simulink model "Schema_Bloc_Instalatie"  (R2017b)
settings: Solver=VariableStepAuto  StartTime=0.0  StopTime=1000  RelTol=1e-3
values from neighbouring files (symbols this model uses):
  k = 0.035    [modelare.m]
  k11 = k2^2+4*(k-k3)*k1    (= 0.0890826)    [modelare.m]
  k12 = 4*(k-k3)*2    (= 0.2848)    [modelare.m]
  k13 = 2*(k-k3)    (= 0.0712)    [modelare.m]
  k2 = -0.015    [modelare.m]
settings Model: Creator=alinvoicu26  LastModifiedBy=alinvoicu26

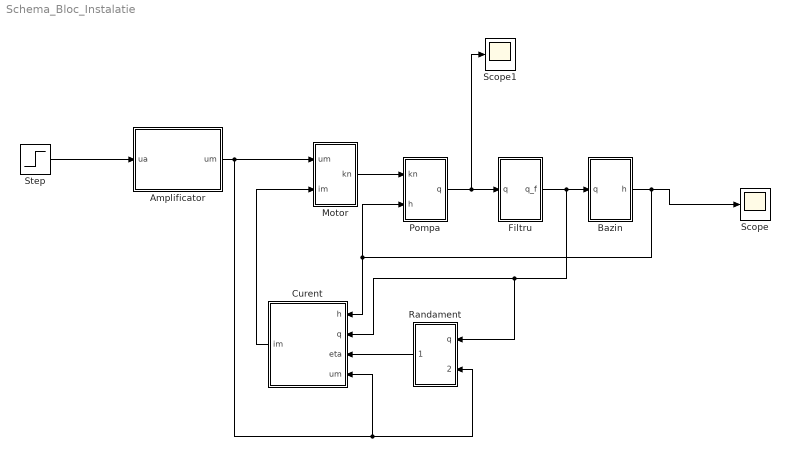
== system Schema_Bloc_Instalatie ==
  Amplificator : Subsystem
  "Bazin " : Subsystem
  Curent : Subsystem
  "Filtru " : Subsystem
  Motor : Subsystem
  "Pompa " : Subsystem
  Randament : Subsystem
  Scope : Scope
  Scope1 : Scope
  Step : Step  After=5  SampleTime=0
  wires:
  Amplificator/1("um ") -> Motor/1(um), Curent/4(um), Randament/2(um)
  Motor/1(kn) -> "Pompa "/1(kn)
  "Pompa "/1("q ") -> Scope1/1, "Filtru "/1("q ")
  "Filtru "/1("q_f ") -> Randament/1(q), Curent/2(q), "Bazin "/1(q)
  "Bazin "/1("h ") -> Curent/1("h "), "Pompa "/2(h), Scope/1
  Randament/1("eta ") -> Curent/3(eta)
  Curent/1("im ") -> Motor/2("im ")
  Step/1 -> Amplificator/1("ua ")

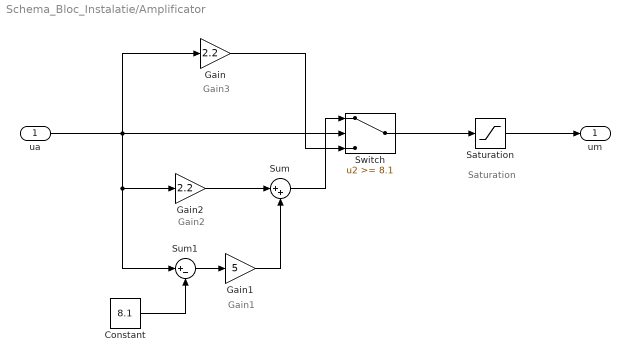
== system Schema_Bloc_Instalatie/Amplificator ==
  note: Saturation
  note: Gain3
  note: Gain2
  note: Gain1
  "ua " : Inport
  Constant : Constant  Value=8.1
  Gain : Gain  Gain=2.2
  Gain1 : Gain  Gain=5
  Gain2 : Gain  Gain=2.2
  Saturation : Saturate  UpperLimit=22  LowerLimit=0
  Sum : Sum  Inputs=|++
  Sum1 : Sum  Inputs=|+-
  Switch : Switch  Threshold=8.1
  "um " : Outport
  wires:
  Switch/1 -> Saturation/1
  Gain2/1 -> Sum/1
  Sum/1 -> Switch/1
  "ua "/1 -> Sum1/1, Gain2/1, Gain/1, Switch/2
  Gain/1 -> Switch/3
  Gain1/1 -> Sum/2
  Sum1/1 -> Gain1/1
  Constant/1 -> Sum1/2
  Saturation/1 -> "um "/1

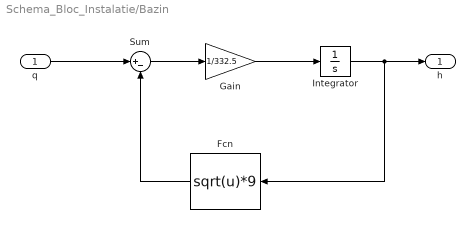
== system Schema_Bloc_Instalatie/Bazin  ==
  q : Inport
  Fcn : Fcn  Expr=sqrt(u)*9
  Gain : Gain  Gain=1/332.5
  Integrator : Integrator
  Sum : Sum  Inputs=|+-
  "h " : Outport
  wires:
  q/1 -> Sum/1
  Fcn/1 -> Sum/2
  Integrator/1 -> Fcn/1, "h "/1
  Gain/1 -> Integrator/1
  Sum/1 -> Gain/1

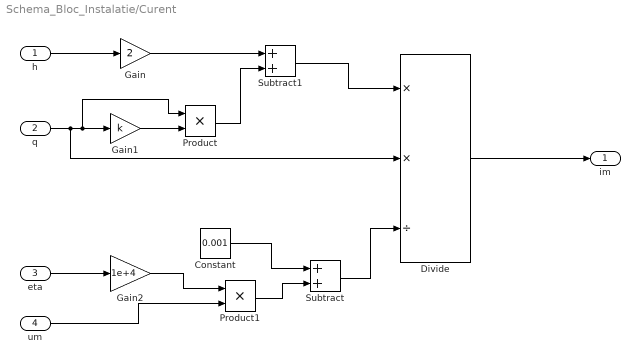
== system Schema_Bloc_Instalatie/Curent ==
  "h " : Inport
  q : Inport  Port=2
  eta : Inport  Port=3
  um : Inport  Port=4
  Constant : Constant  Value=0.001
  Divide : Product  Inputs=**/
  Gain : Gain  Gain=2
  Gain1 : Gain  Gain=k
  Gain2 : Gain  Gain=1e+4
  Product : Product
  Product1 : Product
  Subtract : Sum
  Subtract1 : Sum
  "im " : Outport
  wires:
  Constant/1 -> Subtract/1
  Gain/1 -> Subtract1/1
  q/1 -> Divide/2, Product/1, Gain1/1
  Divide/1 -> "im "/1
  Subtract1/1 -> Divide/1
  Gain2/1 -> Product1/1
  "h "/1 -> Gain/1
  Product1/1 -> Subtract/2
  Subtract/1 -> Divide/3
  eta/1 -> Gain2/1
  Product/1 -> Subtract1/2
  um/1 -> Product1/2
  Gain1/1 -> Product/2

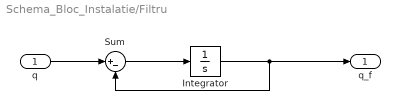
== system Schema_Bloc_Instalatie/Filtru  ==
  "q " : Inport
  Integrator : Integrator
  Sum : Sum  Inputs=|+-
  "q_f " : Outport
  wires:
  Sum/1 -> Integrator/1
  "q "/1 -> Sum/1
  Integrator/1 -> "q_f "/1, Sum/2

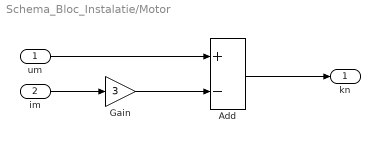
== system Schema_Bloc_Instalatie/Motor ==
  um : Inport
  "im " : Inport  Port=2
  Add : Sum  Inputs=+-
  Gain : Gain  Gain=3
  kn : Outport
  wires:
  "im "/1 -> Gain/1
  Add/1 -> kn/1
  Gain/1 -> Add/2
  um/1 -> Add/1

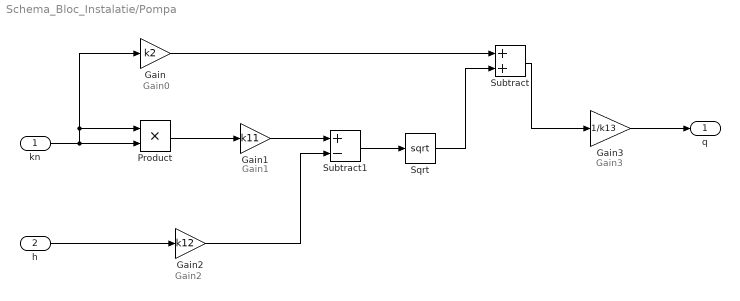
== system Schema_Bloc_Instalatie/Pompa  ==
  note: Gain3
  note: Gain0
  note: Gain2
  note: Gain1
  kn : Inport
  h : Inport  Port=2
  Gain : Gain  Gain=k2
  Gain1 : Gain  Gain=k11
  Gain2 : Gain  Gain=k12
  Gain3 : Gain  Gain=1/k13
  Product : Product
  Sqrt : Sqrt  SaturateOnIntegerOverflow=on
  Subtract : Sum
  Subtract1 : Sum  Inputs=+-
  "q " : Outport
  wires:
  kn/1 -> Product/1, Gain/1, Product/2
  Product/1 -> Gain1/1
  Sqrt/1 -> Subtract/2
  Gain/1 -> Subtract/1
  Subtract/1 -> Gain3/1
  Gain2/1 -> Subtract1/2
  Gain1/1 -> Subtract1/1
  Gain3/1 -> "q "/1
  Subtract1/1 -> Sqrt/1
  h/1 -> Gain2/1

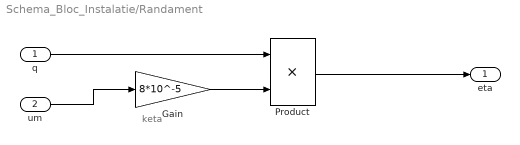
== system Schema_Bloc_Instalatie/Randament ==
  note: keta
  q : Inport
  um : Inport  Port=2
  Gain : Gain  Gain=8*10^-5
  Product : Product
  "eta " : Outport
  wires:
  Gain/1 -> Product/2
  q/1 -> Product/1
  um/1 -> Gain/1
  Product/1 -> "eta "/1
